simulink model "openMHA_test"  (R2020a)
settings: Solver=VariableStepAuto  StartTime=0.0  StopTime=528  RelTol=1e-3
InitFcn:
  | test_init
StopFcn:
  | test_stop
values from neighbouring files (symbols this model uses):
  band_edges = calculate_band_edges(ef, num_bins, binwidth, num_bands)    [test_db_lookup_gain_fpga_init.m]    (also in test_db_lookup_init.m; test_gaintable_init.m; test_init.m; test_state_gainapp_cbuf_init.m = [band_edges mirrored_band_edges])
  num_bins = FFTsize/2 + 1    (= 129)    [test_FFT_to_gain_init.m]    (also in test_ar_filter_gaintable_init.m; test_db_ar_gaintable_init.m; test_db_lookup_gain_fpga_init.m; test_db_lookup_init.m)
undefined symbols (not defined in the file or in its folder): mp
libraries: simulink x3, hdlsllib x3, dspsrcs4 x3
settings Model: Creator=t96f346  LastModifiedBy=t96f346

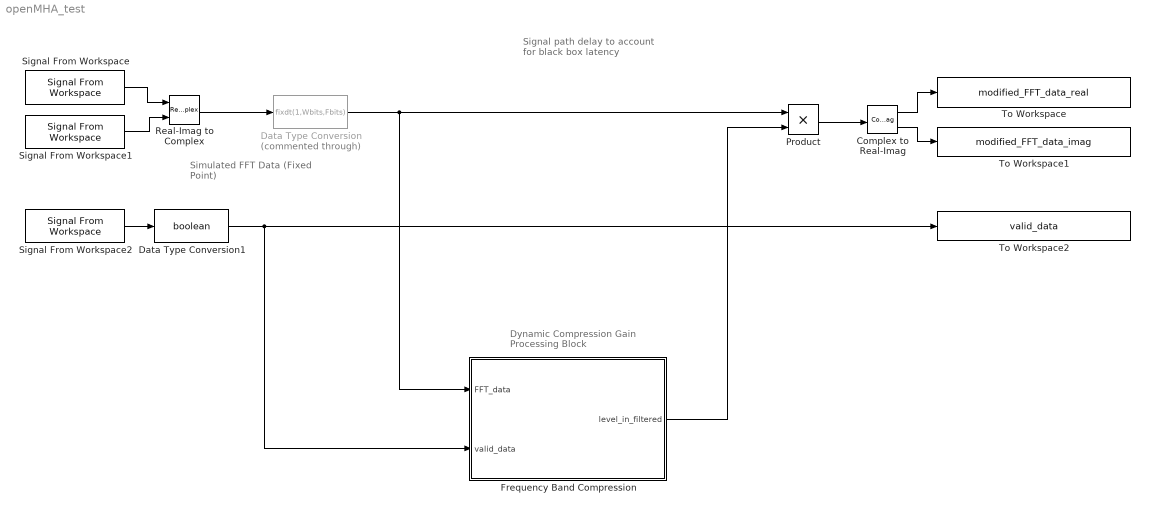
== system openMHA_test ==
  note: Signal path delay to account for black box latency
  note: Simulated FFT Data
      | (Fixed Point)
  note: Dynamic Compression
      | Gain Processing Block
  Complex to Real-Imag : ComplexToRealImag
  Data Type Conversion : DataTypeConversion  Commented=through  OutDataTypeStr=fixdt(1,Wbits,Fbits)
  Data Type Conversion1 : DataTypeConversion  OutDataTypeStr=boolean
  Frequency Band Compression : Subsystem
  Product : Product
  Real-Imag to Complex : RealImagToComplex
  Signal From Workspace : dspsrcs4/Signal From Workspace  X=FFT_data_real  Ts=1  nsamps=1  OutputAfterFinalValue=Setting to zero  ignoreOrWarnInputAndFrameLengths=off  OutputFrames=off
  Signal From Workspace1 : dspsrcs4/Signal From Workspace  X=FFT_data_imag  Ts=1  nsamps=1  OutputAfterFinalValue=Setting to zero  ignoreOrWarnInputAndFrameLengths=off  OutputFrames=off
  Signal From Workspace2 : dspsrcs4/Signal From Workspace  X=valid_data  Ts=1  nsamps=1  OutputAfterFinalValue=Setting to zero  ignoreOrWarnInputAndFrameLengths=off  OutputFrames=off
  To Workspace : ToWorkspace  VariableName=modified_FFT_data_real  SampleTime=-1
      settings: Save2DSignal=2-D array (concatenate along first dimension)
  To Workspace1 : ToWorkspace  VariableName=modified_FFT_data_imag  SampleTime=-1
      settings: Save2DSignal=2-D array (concatenate along first dimension)
  To Workspace2 : ToWorkspace  VariableName=valid_data  SampleTime=-1
      settings: Save2DSignal=2-D array (concatenate along first dimension)
  wires:
  Real-Imag to Complex/1 -> Data Type Conversion/1
  Signal From Workspace1/1 -> Real-Imag to Complex/2
  Signal From Workspace/1 -> Real-Imag to Complex/1
  Frequency Band Compression/1(level_in_filtered) -> Product/2
  Product/1 -> Complex to Real-Imag/1
  Complex to Real-Imag/2 -> To Workspace1/1
  Complex to Real-Imag/1 -> To Workspace/1
  Data Type Conversion/1 -> Frequency Band Compression/1(FFT_data), Product/1
  Signal From Workspace2/1 -> Data Type Conversion1/1
  Data Type Conversion1/1 -> To Workspace2/1, Frequency Band Compression/2(valid_data)

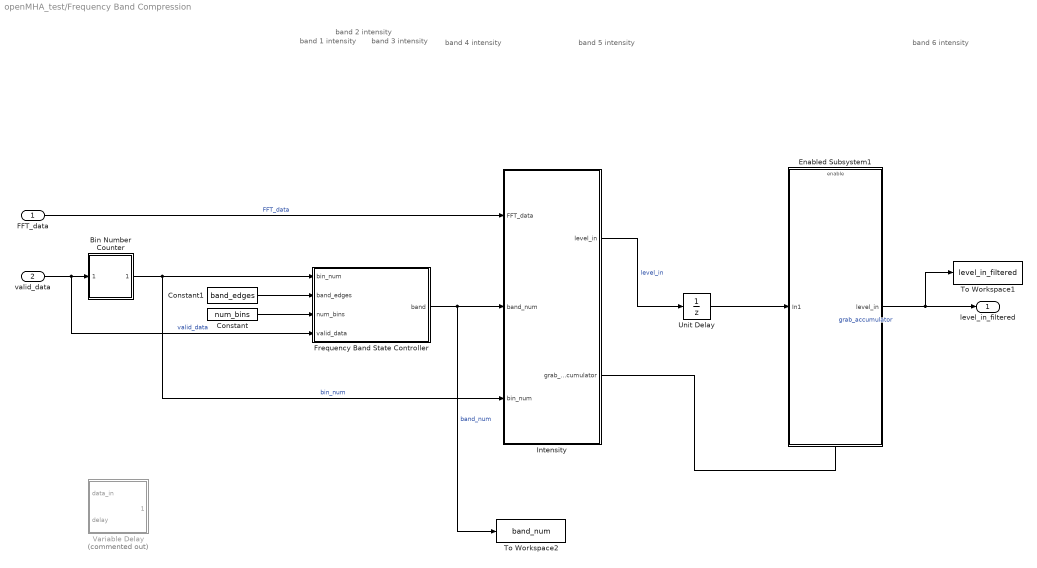
== system openMHA_test/Frequency Band Compression ==
  note: band 1
      | intensity
  note: band 2
      | intensity
  note: band 3
      | intensity
  note: band 4
      | intensity
  note: band 5
      | intensity
  note: band 6
      | intensity
  FFT_data : Inport
  valid_data : Inport  Port=2
  Bin Number Counter : Subsystem
  Constant : Constant  Value=num_bins  SampleTime=-1
  Constant1 : Constant  Value=band_edges  SampleTime=-1
  Enabled Subsystem1 : Subsystem  TreatAsAtomicUnit=on
  Frequency Band State Controller : MATLAB Function  TreatAsAtomicUnit=on
  Intensity : Subsystem
  To Workspace1 : ToWorkspace  VariableName=level_in_filtered  SampleTime=-1
      settings: Save2DSignal=2-D array (concatenate along first dimension)
  To Workspace2 : ToWorkspace  VariableName=band_num  SampleTime=-1
      settings: Save2DSignal=2-D array (concatenate along first dimension)
  Unit Delay : UnitDelay  SampleTime=-1  HasFrameUpgradeWarning=on
  Variable Delay : Subsystem  Commented=on
  level_in_filtered : Outport
  wires:
  FFT_data/1 -> Intensity/1(FFT_data)  "FFT_data"
  valid_data/1 -> Frequency Band State Controller/4(valid_data), Bin Number Counter/1(valid_data)  "valid_data"
  Constant1/1 -> Frequency Band State Controller/2(band_edges)
  Bin Number Counter/1(bin_num) -> Frequency Band State Controller/1(bin_num), Intensity/3(bin_num)  "bin_num"
  Constant/1 -> Frequency Band State Controller/3(num_bins)
  Frequency Band State Controller/1(band) -> To Workspace2/1, Intensity/2(band_num)  "band_num"
  Intensity/1(level_in) -> Unit Delay/1  "level_in"
  Unit Delay/1 -> Enabled Subsystem1/1(In1)
  Intensity/2(grab_accumulator) -> Enabled Subsystem1/Enable  "grab_accumulator"
  Enabled Subsystem1/1(level_in) -> To Workspace1/1, level_in_filtered/1

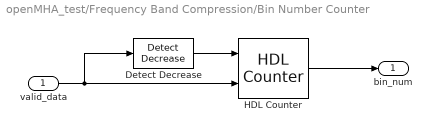
== system openMHA_test/Frequency Band Compression/Bin Number Counter ==
  valid_data : Inport
  Detect Decrease : simulink/Logic and Bit Operations/Detect Decrease  vinit=1  OutDataTypeStr=boolean
  HDL Counter : hdlsllib/Sources/HDL Counter  CountType=Count limited  CountInit=1  CountStep=1  CountMax=num_bins  CountFromType=Initial value  CountFrom=1  CountResetPort=on  CountLoadPort=off  CountEnbPort=on  CountDirPort=off  CountDataType=Unsigned  CountWordLen=8  CountFracLen=0  CountSampTime=1
  bin_num : Outport
  wires:
  valid_data/1 -> HDL Counter/2, Detect Decrease/1
  HDL Counter/1 -> bin_num/1
  Detect Decrease/1 -> HDL Counter/1

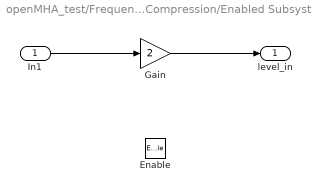
== system openMHA_test/Frequency Band Compression/Enabled Subsystem1 ==
  In1 : Inport
  Enable : EnablePort
  Gain : Gain  Gain=2
  level_in : Outport  InitialOutput=0  VectorParamsAs1DForOutWhenUnconnected=off
  wires:
  In1/1 -> Gain/1
  Gain/1 -> level_in/1

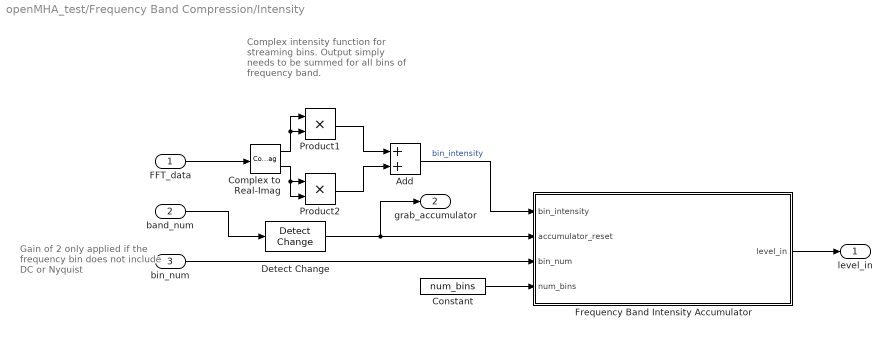
== system openMHA_test/Frequency Band Compression/Intensity ==
  note: Complex intensity function for streaming bins. Output simply needs to be summed for all bins of frequency band.
  note: Gain of 2 only applied if the frequency bin does not include DC or Nyquist
  FFT_data : Inport
  band_num : Inport  Port=2
  bin_num : Inport  Port=3
  Add : Sum
  Complex to Real-Imag : ComplexToRealImag
  Constant : Constant  Value=num_bins  SampleTime=-1
  Detect Change : simulink/Logic and Bit Operations/Detect Change  vinit=0  OutDataTypeStr=boolean
  Frequency Band Intensity Accumulator : MATLAB Function  TreatAsAtomicUnit=on
  Product1 : Product
  Product2 : Product
  level_in : Outport
  grab_accumulator : Outport  Port=2  VectorParamsAs1DForOutWhenUnconnected=off
  wires:
  Product2/1 -> Add/2
  Complex to Real-Imag/1 -> Product1/1, Product1/2
  Complex to Real-Imag/2 -> Product2/2, Product2/1
  Product1/1 -> Add/1
  Add/1 -> Frequency Band Intensity Accumulator/1(bin_intensity)  "bin_intensity"
  FFT_data/1 -> Complex to Real-Imag/1
  Frequency Band Intensity Accumulator/1(level_in) -> level_in/1
  band_num/1 -> Detect Change/1
  Detect Change/1 -> Frequency Band Intensity Accumulator/2(accumulator_reset), grab_accumulator/1
  bin_num/1 -> Frequency Band Intensity Accumulator/3(bin_num)
  Constant/1 -> Frequency Band Intensity Accumulator/4(num_bins)

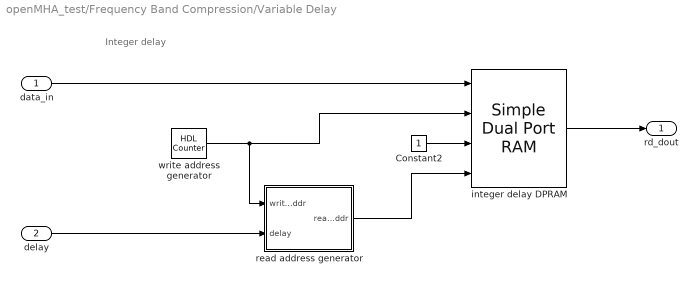
== system openMHA_test/Frequency Band Compression/Variable Delay ==
  note: Integer delay
  data_in : Inport
  delay : Inport  Port=2
  Constant2 : Constant  OutDataTypeStr=Inherit: Inherit via back propagation  SampleTime=-1
  integer delay DPRAM : hdlsllib/HDL RAMs/Simple Dual Port RAM  ram_size=mp.integerDelayAddrSize
      settings: SourceProductBaseCode=SL
  read address generator : Subsystem
  write address generator : hdlsllib/Sources/HDL Counter  CountType=Count limited  CountInit=0  CountStep=1  CountMax=mp.integerDelayBufferSize - 1  CountFromType=Initial value  CountFrom=0  CountResetPort=off  CountLoadPort=off  CountEnbPort=off  CountDirPort=off  CountDataType=Unsigned  CountWordLen=mp.integerDelayAddrSize  CountFracLen=0  CountSampTime=mp.Ts
  rd_dout : Outport
  wires:
  read address generator/1(read_addr) -> integer delay DPRAM/4
  integer delay DPRAM/1 -> rd_dout/1
  write address generator/1 -> read address generator/1(write_addr), integer delay DPRAM/2
  delay/1 -> read address generator/2(delay)
  Constant2/1 -> integer delay DPRAM/3
  data_in/1 -> integer delay DPRAM/1

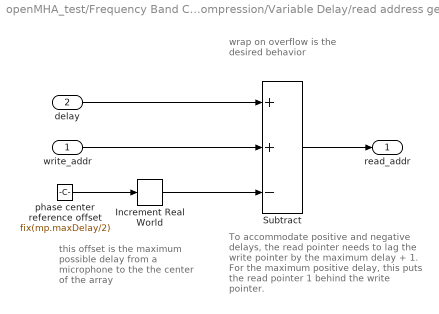
== system openMHA_test/Frequency Band Compression/Variable Delay/read address generator ==
  note: wrap on overflow is the desired behavior
  note: this offset is the maximum possible delay from a microphone to the the center of the array
  note: To accommodate positive and negative delays, the read pointer needs to lag the write pointer by the maximum delay + 1. For the maximum positive delay, this puts the read pointer 1 behind the write pointer.
  write_addr : Inport
  delay : Inport  Port=2
  Increment Real World : simulink/Additional Math & Discrete/Additional Math: Increment - Decrement/Increment Real World
      settings: SourceProductBaseCode=SL
  Subtract : Sum  Inputs=++-  OutDataTypeStr=Inherit: Inherit via back propagation
  phase center reference offset : Constant  Value=fix(mp.maxDelay/2)  OutDataTypeStr=fixdt(0,delayDataTypeWordLength - delayDataTypeFractionLength,0)  SampleTime=-1
  read_addr : Outport  VectorParamsAs1DForOutWhenUnconnected=off
  wires:
  Subtract/1 -> read_addr/1
  Increment Real World/1 -> Subtract/3
  phase center reference offset/1 -> Increment Real World/1
  write_addr/1 -> Subtract/2
  delay/1 -> Subtract/1

== matlab function openMHA_test/Frequency Band Compression/Frequency Band State Controller ==
  data: bin_num input; band output; band_edges input size=[1 32]; num_bins input; valid_data input
%#codegen
function band = band_state(bin_num, band_edges, num_bins, valid_data)
% Moore State Machine

%------------------------------------------------------------------------%
% The following is a Moore State Machine in which each state represents the
% frequency band in which the dynamic compression model is operating. The
% frequency bin number or index is the input to the state machine and
% determines whether whether the next state will be in the current or next
% frequency band. The band_edges input is designed to read from a
% precomputed band edge index vector, which sets the boundaries between
% each frequency band and serves as the conditional value.
%------------------------------------------------------------------------%

% y = f(x) : 
% all actions are state actions and 
% outputs are pure functions of state only 

% Defining All Possible Frequency Band States
fb1 = 1;
fb2 = 2;
fb3 = 3;
fb4 = 4;
fb5 = 5;
fb6 = 6;
fb7 = 7;
fb8 = 8;
fb9 = 9;
fb10 = 10;
fb11 = 11;
fb12 = 12;
fb13 = 13;
fb14 = 14;
fb15 = 15;
fb16 = 16;
fb17 = 17;
fb18 = 18;
fb19 = 19;
fb20 = 20;
fb21 = 21;
fb22 = 22;
fb23 = 23;
fb24 = 24;
fb25 = 25;
fb26 = 26;
fb27 = 27;
fb28 = 28;
fb29 = 29;
fb30 = 30;
fb31 = 31;
fb32 = 32;


% Using persistent keyword to model state registers in hardware
persistent curr_state;
if isempty(curr_state)
    curr_state = fb1;   
end

% Switch to new state (frequency band) based on the value state register
switch (curr_state)
    
    case fb1
        
        % value of output band depends only on state and not on inputs
        band = uint8(1);
        
        % decide next state value based on inputs
        if (bin_num >= num_bins) 
            curr_state = fb1;
        elseif (bin_num >= band_edges(band)) && (valid_data == true)
            curr_state = fb2;
        else
            curr_state = fb1;
        end
        
    case fb2
        
        band = uint8(2);
        
        if (bin_num >= num_bins)
            curr_state = fb1;
        elseif (bin_num >= band_edges(band))
            curr_state = fb3;
        else
            curr_state = fb2;
        end
        
    case fb3
        
        band = uint8(3);
        
        if (bin_num >= num_bins)
            curr_state = fb1;
        elseif (bin_num >= band_edges(band))
            curr_state = fb4;
        else
            curr_state = fb3;
        end
        
    case fb4
        
        band = uint8(4);
        
        if (bin_num >= num_bins)
            curr_state = fb1;
        elseif (bin_num >= band_edges(band))
            curr_state = fb5;
        else
            curr_state = fb4;
        end
        
    case fb5
        
        band = uint8(5);
        
        if (bin_num >= num_bins)
            curr_state = fb1;
        elseif (bin_num >= band_edges(band))
            curr_state = fb6;
        else
            curr_state = fb5;
        end
        
    case fb6
        
        band = uint8(6);
        
        if (bin_num >= num_bins)
            curr_state = fb1;
        elseif (bin_num >= band_edges(band))
            curr_state = fb7;
        else
            curr_state = fb6;
        end
        
    case fb7
        
        band = uint8(7);
        
        if (bin_num >= num_bins)
            curr_state = fb1;
        elseif (bin_num >= band_edges(band))
            curr_state = fb8;
        else
            curr_state = fb7;
        end
        
    case fb8
        
        band = uint8(8);
        
        if (bin_num >= num_bins)
            curr_state = fb1;
        elseif (bin_num >= band_edges(band))
            curr_state = fb9;
        else
            curr_state = fb8;
        end
        
    case fb9
        
        band = uint8(9);
        
        if (bin_num >= num_bins)
            curr_state = fb1;
        elseif (bin_num >= band_edges(band))
            curr_state = fb10;
        else
            curr_state = fb9;
        end
        
    case fb10
        
        band = uint8(10);
        
        if (bin_num >= num_bins)
            curr_state = fb1;
        elseif (bin_num >= band_edges(band))
            curr_state = fb11;
        else
            curr_state = fb10;
        end
        
    case fb11
        
        band = uint8(11);
        
        if (bin_num >= num_bins)
            curr_state = fb1;
        elseif (bin_num >= band_edges(band))
            curr_state = fb12;
        else
            curr_state = fb11;
        end
        
    case fb12
        
        band = uint8(12);
        
        if (bin_num >= num_bins)
            curr_state = fb1;
        elseif (bin_num >= band_edges(band))
            curr_state = fb13;
        else
            curr_state = fb12;
        end
        
    case fb13
        
        band = uint8(13);
        
        if (bin_num >= num_bins)
            curr_state = fb1;
        elseif (bin_num >= band_edges(band))
            curr_state = fb14;
        else
            curr_state = fb13;
        end
      
    case fb14
        
        band = uint8(14);
        
        if (bin_num >= num_bins)
            curr_state = fb1;
        elseif (bin_num >= band_edges(band))
            curr_state = fb15;
        else
            curr_state = fb14;
        end
        
    case fb15
        
        band = uint8(15);
        
        if (bin_num >= num_bins)
            curr_state = fb1;
        elseif (bin_num >= band_edges(band))
            curr_state = fb16;
        else
            curr_state = fb15;
        end
        
    case fb16
        
        band = uint8(16);
        
        if (bin_num >= num_bins)
            curr_state = fb1;
        elseif (bin_num >= band_edges(band))
            curr_state = fb17;
        else
            curr_state = fb16;
        end
        
    case fb17
        
        band = uint8(17);
        
        if (bin_num >= num_bins)
            curr_state = fb1;
        elseif (bin_num >= band_edges(band))
            curr_state = fb18;
        else
            curr_state = fb17;
        end
        
    case fb18
        
        band = uint8(18);
        
        if (bin_num >= num_bins)
            curr_state = fb1;
        elseif (bin_num >= band_edges(band))
            curr_state = fb19;
        else
            curr_state = fb18;
        end
        
    case fb19
        
        band = uint8(19);
        
        if (bin_num >= num_bins)
            curr_state = fb1;
        elseif (bin_num >= band_edges(band))
            curr_state = fb20;
        else
            curr_state = fb19;
        end
        
    case fb20
        
        band = uint8(20);
        
        if (bin_num >= num_bins)
            curr_state = fb1;
        elseif (bin_num >= band_edges(band))
            curr_state = fb21;
        else
            curr_state = fb20;
        end
        
    case fb21
        
        band = uint8(21);
        
        if (bin_num >= num_bins)
            curr_state = fb1;
        elseif (bin_num >= band_edges(band))
            curr_state = fb22;
        else
            curr_state = fb21;
        end
        
    case fb22
        
        band = uint8(22);
        
        if (bin_num >= num_bins)
            curr_state = fb1;
        elseif (bin_num >= band_edges(band))
            curr_state = fb23;
        else
            curr_state = fb22;
        end
        
    case fb23
        
        band = uint8(23);
        
        if (bin_num >= num_bins)
            curr_state = fb1;
        elseif (bin_num >= band_edges(band))
            curr_state = fb24;
        else
            curr_state = fb23;
        end
        
    case fb24
        
        band = uint8(24);
        
        if (bin_num >= num_bins)
            curr_state = fb1;
        elseif (bin_num >= band_edges(band))
            curr_state = fb25;
        else
            curr_state = fb24;
        end
        
    case fb25
        
        band = uint8(25);
        
        if (bin_num >= num_bins)
            curr_state = fb1;
        elseif (bin_num >= band_edges(band))
            curr_state = fb26;
        else
            curr_state = fb25;
        end
        
    case fb26
        
        band = uint8(26);
        
        if (bin_num >= num_bins)
            curr_state = fb1;
        elseif (bin_num >= band_edges(band))
            curr_state = fb27;
        else
            curr_state = fb26;
        end
        
    case fb27
        
        band = uint8(27);
        
        if (bin_num >= num_bins)
            curr_state = fb1;
        elseif (bin_num >= band_edges(band))
            curr_state = fb28;
        else
            curr_state = fb27;
        end
        
    case fb28
        
        band = uint8(28);
        
        if (bin_num >= num_bins)
            curr_state = fb1;
        elseif (bin_num >= band_edges(band))
            curr_state = fb29;
        else
            curr_state = fb28;
        end
        
    case fb29
        
        band = uint8(29);
        
        if (bin_num >= num_bins)
            curr_state = fb1;
        elseif (bin_num >= band_edges(band))
            curr_state = fb30;
        else
            curr_state = fb29;
        end
        
    case fb30
        
        band = uint8(30);
        
        if (bin_num >= num_bins)
            curr_state = fb1;
        elseif (bin_num >= band_edges(band))
            curr_state = fb31;
        else
            curr_state = fb30;
        end
        
    case fb31
        
        band = uint8(31);
        
        if (bin_num >= num_bins)
            curr_state = fb1;
        elseif (bin_num >= band_edges(band))
            curr_state = fb32;
        else
            curr_state = fb31;
        end
        
    case fb32
        
        band = uint8(32);
        
        if (bin_num >= num_bins)
            curr_state = fb1;
        elseif (bin_num >= band_edges(band))
            curr_state = fb1;
        else
            curr_state = fb32;
        end
        
    otherwise
        band = uint8(1);
        
end

== matlab function openMHA_test/Frequency Band Compression/Intensity/Frequency Band Intensity Accumulator ==
  data: bin_intensity input; level_in output; accumulator_reset input; bin_num input; num_bins input
function level_in = accumulate_band(bin_intensity, accumulator_reset, bin_num, num_bins)

% Accumulates the bin intensities until a new frequency band is detected.
% Takes in the current frequency bin intensity, an accumulator reset
% control signal, bin number and number of frequency bins. If the 
% accumulator_reset is true, the sum is reset starting with the current 
% frequency bin intensity. Unless a DC or Nyquist bin is detected, a
% logical shift left is executed to apply a gain of two to the current
% bin_intensity, which accounts for negative frequencies.

persistent total;

if isempty(total)
    total = 0;
end

if bin_num == 1 || bin_num == num_bins
    dc_nyquist = true;
else
    dc_nyquist = false;
end

if accumulator_reset == true && dc_nyquist == true
    total = bin_intensity;
    level_in = total;
elseif accumulator_reset == true && dc_nyquist == false
    total = bitsll(bin_intensity,fi(1));
    level_in = total;
elseif accumulator_reset == false && dc_nyquist == true
    total = total + bin_intensity;
    level_in = total;
elseif accumulator_reset == false && dc_nyquist == false
    total = total + bitsll(bin_intensity,fi(1));
    level_in = total;
else
    total = inf;
    error('Incorrect Logic in accumulate_band function!');
end
